simulink model "analog_integrator"  (R2020b)
settings: Solver=ode1be  StartTime=0.0  StopTime=30  RelTol=1e-3  AbsTol=1e-3
libraries: analogCompBlocks x4, ee_lib x2, fl_lib x1, nesl_utility x1
settings Model: DataDictionary=analogComputerData.sldd  EnableAccessToBaseWorkspace=off  OrderedModelArguments=off  Creator=roadrunner  LastModifiedBy=roadrunner
settings SolverCC: AutoScaleAbsTol=off
settings DebuggingCC: SymbolicDimsDataTypeCodeGenerationDiagnostic=none
settings SFSimCC: CustomCodeUndefinedFunction=UseInterfaceOnly
settings SimscapeCC: SimscapeLogType=all  SimscapeLogSimulationStatistics=on  SimscapeLogDataHistory=10000

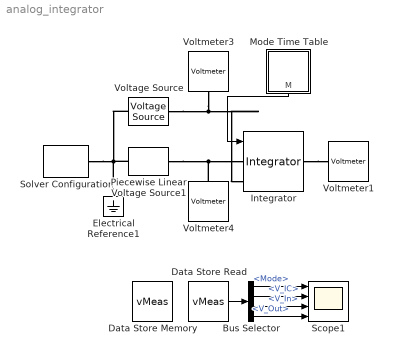
== system analog_integrator ==
  Bus Selector : BusSelector  OutputSignals=Mode,V_IC,V_In,V_Out
  Data Store Memory : DataStoreMemory  Priority=5  DataStoreName=vMeas  ReadBeforeWriteMsg=warning  WriteAfterWriteMsg=warning  WriteAfterReadMsg=warning  ShowAdditionalParam=off  OutDataTypeStr=Bus: bus_integrator_measurements
  Data Store Read : DataStoreRead  Priority=6  DataStoreName=vMeas
  Electrical Reference1 : fl_lib/Electrical/Electrical Elements/Electrical Reference
  Integrator : analogCompBlocks/Integrator  capacitance=0.01  small_resistance=0.01  tau=1
  Mode Time Table : Subsystem  Priority=0  mask{DSNAME='vMeas', DSELEMENT='Mode'}
      mask prompts: DSNAME "Data Store Name"; DSELEMENT "Data Store Element"
      mask init:
      | % Set data store name
      | DSBLOCK = [gcb '/DataStoreWrite'];
      | set_param(DSBLOCK,'DataStoreName',DSNAME)
      | 
      | % Set data store write element
      | DSELEMENT = [DSNAME '.' DSELEMENT];
      | set_param(DSBLOCK,'DataStoreElements',DSELEMENT)
      settings: AttributesFormatString=Mode Time Table
  Piecewise Linear Voltage Source1 : ee_lib/Additional Components/SPICE Sources/Piecewise Linear Voltage Source  TIMElist=[10 10.01 15 15.01 20 20.01] s  VOLTlist=[0 -1 -1 1 1 0] V  INTERP=1  EXTRAP=2
      settings: AttributesFormatString=Voltage In  SourceProductBaseCode=PS  InternalSimscapePortConfiguration="{\"Bottom\":[],\"Left\":[{\"id\":\"p\",\"label\":\"+\",\"type\":\"foundation.electrical.electrical\"}],\"Right\":[{\"id\":\"n\",\"label\":\"-\",\"type\":\"foundation.electrical.electrical\"}],\"Top\":[]}"
  Scope1 : Scope  NumInputPorts=4
  Solver Configuration : nesl_utility/Solver Configuration  PhysicalDomain=network_engine_domain  SubClassName=solver  LeftPortType=input  RightPortType=generic  Tones=[]  Harmonics=[]  SimulateNoise=off  Profile=off  UseLocalSampling=off  EnableSwitchedLinearOptims=on  FrequencyDomain=off  UseCCode=off  RelTol=0.001  AbsTol=1e-06  MinStep=1e-09  ToWorkspace=off  RevertToSquareIcSolve=off  NumHomotopyIterations=100  PhasorMode=off  PhasorModeNumHarmonics=1  DoDC=off  ResidualTolerance=1e-09  UseLocalSolver=on  LocalSolverChoice=NE_BACKWARD_EULER_ADVANCER  LocalSolverSampleTime=0.01  DoFixedCost=on  MaxNonlinIter=3  MaxModeIter=2  ComputeImpulses=off  ImpulseIterations=2  LinearAlgebra=auto  EquationFormulation=NE_TIME_EF  DelaysMemoryBudget=1024  AutomaticFiltering=on  FilteringTimeConstant=0.001  PartitionStorageMethod=AS_NEEDED  PartitionMemoryBudget=1024  PartitionMethod=ROBUST
      settings: SourceProductName=Utilities
  Voltage Source : ee_lib/Sources/Voltage Source  dc_voltage=10 V  ac_voltage=0 V  ac_shift=0 rad  ac_frequency=60 Hz  noise_mode=0  PSD=0 V^2/Hz  repeatability=1  auto_seed=4251255130  user_seed=0  sample_time=1e-3 s  i_specify=off  i_priority=None  i=0 A  i_nominal_specify=off  i_nominal_unit=A  i_nominal_value=1  v_specify=off  v_priority=None  v=0 V  v_nominal_specify=off  v_nominal_unit=V  v_nominal_value=1
      settings: AttributesFormatString=Voltage IC
  Voltmeter1 : analogCompBlocks/Voltmeter  Priority=4  DSNAME='vMeas'  DSELEMENT='V_Out'
      settings: AttributesFormatString=Voltage Sensor
  Voltmeter3 : analogCompBlocks/Voltmeter  Priority=1  DSNAME='vMeas'  DSELEMENT='V_IC'
      settings: AttributesFormatString=Voltage Sensor
  Voltmeter4 : analogCompBlocks/Voltmeter  Priority=2  DSNAME='vMeas'  DSELEMENT='V_In'
      settings: AttributesFormatString=Voltage Sensor
  wires:
  Data Store Read/1 -> Bus Selector/1
  Mode Time Table/1(M) -> Integrator/1
  Bus Selector/1 -> Scope1/1  "<Mode>"
  Bus Selector/2 -> Scope1/2  "<V_IC>"
  Bus Selector/3 -> Scope1/3  "<V_In>"
  Bus Selector/4 -> Scope1/4  "<V_Out>"
  connections:
  Electrical Reference1/LConn1 -- Piecewise Linear Voltage Source1/RConn1 -- Voltage Source/RConn1 -- Solver Configuration/RConn1
  Piecewise Linear Voltage Source1/LConn1 -- Integrator/LConn1 -- Voltmeter4/LConn1
  Voltage Source/LConn1 -- Integrator/LConn2 -- Voltmeter3/LConn1
  Integrator/RConn1 -- Voltmeter1/LConn1

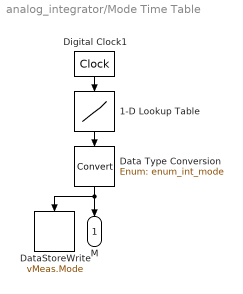
== system analog_integrator/Mode Time Table ==
  1-D Lookup Table : Lookup_n-D  NumberOfTableDimensions=1  BreakpointsForDimension1=[0 5 10 20]  Table=[1 0 2 1]  InterpMethod=Flat  ExtrapMethod=Clip  InternalRulePriority=Speed  OutDataTypeStr=int32  RndMeth=Simplest  InputSameDT=on
      settings: AttributesFormatString=|
      | Integrator Mode
      | Time Table
  Data Type Conversion : DataTypeConversion  OutDataTypeStr=Enum: enum_int_mode
      settings: AttributesFormatString=|
      | Convert to
      | Mode Enum
  DataStoreWrite : DataStoreWrite  DataStoreName=vMeas  DataStoreElements=vMeas.Mode
  Digital Clock1 : DigitalClock  SampleTime=0.01
      settings: AttributesFormatString=Timer
  M : Outport
  wires:
  1-D Lookup Table/1 -> Data Type Conversion/1
  Digital Clock1/1 -> 1-D Lookup Table/1
  Data Type Conversion/1 -> DataStoreWrite/1, M/1
